simulink model "Tail_sitter_aut1_2016a"  (R2016a)
settings: Solver=ode4  StartTime=0.0  StopTime=13  FixedStep=0.02  RelTol=1e-3
settings Model: Creator=EA-IS  LastModifiedBy=EAIN
settings DebuggingCC: SFUnexpectedBacktrackingDiag=error  SFNoUnconditionalDefaultTransitionDiag=error
settings GRTTargetCC: TargetLangStandard=C99 (ISO)  GeneratePreprocessorConditionals=Use local settings
settings ConfigComp: CovMetricSettings=dwe  CovHtmlReporting=off  CovSaveCumulativeToWorkspaceVar=off  CovSaveSingleToWorkspaceVar=off  CovExternalEMLEnable=on

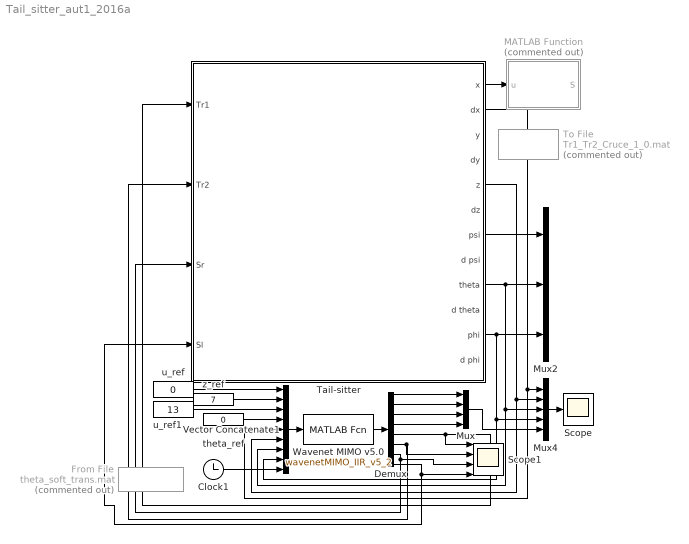
== system Tail_sitter_aut1_2016a ==
  Clock1 : Clock
  Demux : Demux  Outputs=8
  From File : FromFile  Commented=on  FileName=theta_soft_trans.mat  SampleTime=0
  MATLAB Function : MATLAB Function  Commented=on  TreatAsAtomicUnit=on
  Mux : Mux
  Mux2 : Mux  Inputs=3
  Mux4 : Mux  Inputs=5
  Scope : Scope
  Scope1 : Scope  NumInputPorts=4
  "Tail-sitter " : Subsystem
  To File : ToFile  Commented=on  Filename=Tr1_Tr2_Cruce_1_0.mat  SaveFormat=Timeseries
  Vector Concatenate1 : Concatenate  NumInputs=9
  "Wavenet MIMO v5.0 " : MATLABFcn  MATLABFcn=wavenetMIMO_IIR_v5_2  OutputDimensions=8
  theta_ref : Constant  Value=0
  u_ref : Constant  Value=0
  u_ref1 : Constant  Value=13
  z_ref : Constant  Value=7
  wires:
  "Tail-sitter "/7(psi) -> Mux2/1
  Clock1/1 -> Vector Concatenate1/9
  "Tail-sitter "/2(dx) -> Mux4/1, Vector Concatenate1/5
  "Wavenet MIMO v5.0 "/1 -> Demux/1
  "Tail-sitter "/9(theta) -> Mux2/2, Mux4/3, Vector Concatenate1/7
  "Tail-sitter "/11(phi) -> Mux2/3, Mux4/4, Vector Concatenate1/8
  Demux/4 -> Mux/4
  Demux/3 -> Mux/3
  Demux/2 -> Mux/2
  Demux/1 -> Mux/1
  theta_ref/1 -> Vector Concatenate1/4
  "Tail-sitter "/5(z) -> Mux4/2, Vector Concatenate1/6
  z_ref/1 -> Vector Concatenate1/2
  u_ref/1 -> Vector Concatenate1/1
  Mux/1 -> Mux4/5
  Demux/5 -> Scope1/1, "Tail-sitter "/1(Tr1)
  Demux/6 -> Scope1/2, "Tail-sitter "/2("Tr2 ")
  Demux/7 -> Scope1/3, "Tail-sitter "/3(Sr)
  Demux/8 -> Scope1/4, "Tail-sitter "/4("Sl ")
  Vector Concatenate1/1 -> "Wavenet MIMO v5.0 "/1
  u_ref1/1 -> Vector Concatenate1/3
  Mux4/1 -> Scope/1
  "Tail-sitter "/1(x) -> MATLAB Function/1(u)

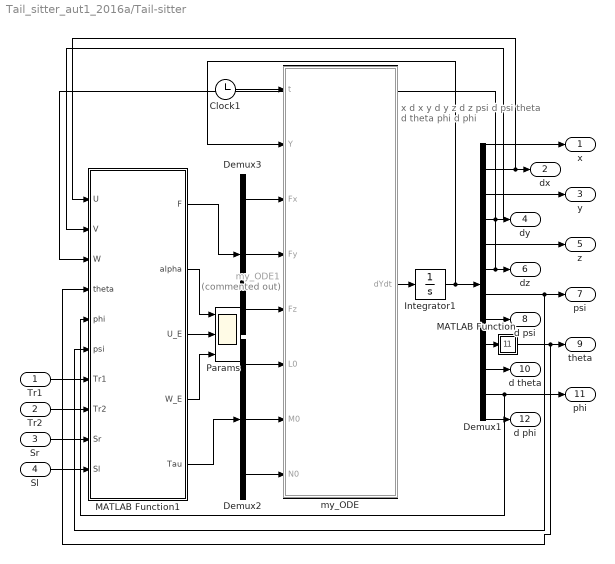
== system Tail_sitter_aut1_2016a/Tail-sitter  ==
  note: x
      |   d x
      |    y
      |   d y
      |    z
      |   d z
      |   psi
      |  d psi
      |  theta
      | d theta
      |   phi
      |  d phi
  Tr1 : Inport
  "Tr2 " : Inport  Port=2
  Sr : Inport  Port=3
  "Sl " : Inport  Port=4
  Clock1 : Clock
  Demux1 : Demux  Outputs=12
  Demux2 : Demux  Outputs=3
  Demux3 : Demux  Outputs=3
  Integrator1 : Integrator  InitialCondition=[0,8.0,0,0,18.0,0,0,0,-pi()/1.97,0,0,0]  UpperSaturationLimit=55  LowerSaturationLimit=-55
  MATLAB Function : MATLAB Function  TreatAsAtomicUnit=on
  MATLAB Function1 : MATLAB Function  TreatAsAtomicUnit=on
  Params : Scope  NumInputPorts=3
  my_ODE : MATLAB Function  TreatAsAtomicUnit=on
  my_ODE1 : MATLAB Function  Commented=on  TreatAsAtomicUnit=on
  x : Outport
  dx : Outport  Port=2
  y : Outport  Port=3
  dy : Outport  Port=4
  z : Outport  Port=5
  dz : Outport  Port=6
  psi : Outport  Port=7
  d psi : Outport  Port=8
  theta : Outport  Port=9
  d theta : Outport  Port=10
  phi : Outport  Port=11
  "d phi " : Outport  Port=12
  wires:
  Demux1/7 -> psi/1, MATLAB Function1/6(psi)
  Demux1/11 -> phi/1, MATLAB Function1/5(phi)
  "Sl "/1 -> MATLAB Function1/10(Sl)
  Demux1/9 -> MATLAB Function/1(theta_rad)
  Demux1/10 -> d theta/1
  Demux1/2 -> MATLAB Function1/1(U), dx/1
  Demux1/8 -> d psi/1
  Demux1/4 -> MATLAB Function1/2(V), dy/1
  Demux1/6 -> MATLAB Function1/3(W), dz/1
  Demux1/3 -> y/1
  Demux1/12 -> "d phi "/1
  Demux1/1 -> x/1
  "Tr2 "/1 -> MATLAB Function1/8(Tr2)
  Sr/1 -> MATLAB Function1/9(Sr)
  Tr1/1 -> MATLAB Function1/7(Tr1)
  Demux1/5 -> z/1
  Demux2/3 -> my_ODE/8(N0)
  Demux2/2 -> my_ODE/7(M0)
  Demux2/1 -> my_ODE/6(L0)
  Demux3/2 -> my_ODE/4(Fy)
  Demux3/1 -> my_ODE/3(Fx)
  Clock1/1 -> my_ODE/1(t)
  my_ODE/1(dYdt) -> Integrator1/1
  Integrator1/1 -> Demux1/1, my_ODE/2(Y)
  Demux3/3 -> my_ODE/5(Fz)
  MATLAB Function1/1(F) -> Demux3/1
  MATLAB Function1/2(alpha) -> Params/1
  MATLAB Function1/3(U_E) -> Params/2
  MATLAB Function1/4(W_E) -> Params/3
  MATLAB Function1/5(Tau) -> Demux2/1
  MATLAB Function/1(theta) -> MATLAB Function1/4(theta), theta/1

== matlab function Tail_sitter_aut1_2016a/MATLAB Function ==
  data: u input; S output
function S = fcn(u)
%S=-40.735;
S=0.4*sin(u)+4;

== matlab function Tail_sitter_aut1_2016a/Tail-sitter /my_ODE ==
  data: t input; dYdt output; Y input; Fx input; Fy input; Fz input; L0 input; M0 input; N0 input
function dYdt = my_ODE(t,Y,Fx,Fy,Fz,L0,M0,N0)
%#codegen

%    This function was generated by the Symbolic Math Toolbox version 8.1.
%    02-Oct-2021 14:11:46

t4 = Y(9);
t2 = cos(t4);
t6 = Y(11);
t3 = cos(t6);
t5 = t2.^2;
t7 = t3.^2;
t8 = sin(t6);
t9 = sin(t4);
t10 = t9.^2;
t11 = t8.^2;
t12 = Y(10);
t13 = Y(12);
t14 = t12.^2;
t15 = Y(8);
t16 = t13.^2;
t17 = t6.*2.0;
t18 = sin(t17);
t19 = t15.^2;
t20 = t7.^2;
t21 = t4.*2.0;
t22 = sin(t21);
t23 = t5.*t20.*4.595542888221475e54;
t24 = t5.*4.407732460960101e54;
t25 = t7.*4.657144927034328e54;
t26 = t10.*5.77375154539186e54;
t27 = t11.*1.244230110983038e49;
t28 = t5.*t7.*t11.*4.595542888221475e54;
t32 = t5.*t7.*9.252684871516254e54;
t33 = t5.*t11.*9.498561560829538e48;
t34 = t7.*t10.*4.657144927034328e54;
t35 = t10.*t11.*1.244230110983038e49;
t29 = t23+t24+t25+t26+t27+t28-t32-t33-t34-t35-5.77375154539186e54;
t30 = 1.0./t29;
t31 = t5.^2;
dYdt = [Y(2);Fx.*(5.0e1./4.9e1);Y(4);Fy.*(5.0e1./4.9e1);Y(6);Fz.*(5.0e1./4.9e1)-9.81e2./1.0e2;t15;t30.*(L0.*3.276779764924493e59-L0.*t7.*2.643071517583136e59-L0.*t11.*7.06138464484666e53+N0.*t9.*3.276779764924493e59-N0.*t2.*t3.*5.32043137111061e56-N0.*t7.*t9.*2.643071517583136e59-N0.*t9.*t11.*7.06138464484666e53-t2.*t8.*t14.*1.919939909312306e55+t2.*t8.*t16.*1.919939909312306e55+t2.*t12.*t13.*1.563784160774438e56-t3.*t12.*t15.*3.839879818624611e55+t9.*t14.*t18.*5.834132374442543e57-t12.*t15.*t22.*9.027036080046288e57+M0.*t2.*t3.*t8.*2.643064456198491e59+N0.*t2.*t3.*t7.*4.291493974897115e56+N0.*t2.*t3.*t11.*4.291493974897115e56+t2.*t7.*t8.*t14.*1.54863581132113e55-t2.*t7.*t8.*t16.*4.137426121757868e49+t2.*t7.*t12.*t13.*2.321039366712225e58-t3.*t8.*t9.*t14.*1.166826474888509e58+t2.*t8.*t11.*t14.*4.137426121757868e49+t3.*t5.*t12.*t15.*3.86527061966559e55+t2.*t7.*t8.*t19.*1.548631673895008e55-t2.*t3.*t14.*t18.*9.472745541356636e54-t2.*t8.*t11.*t16.*4.137426121757868e49+t3.*t7.*t12.*t15.*3.09727162264226e55+t2.*t9.*t12.*t15.*2.349290791384762e58-t2.*t11.*t12.*t13.*3.369918716829444e50+t2.*t8.*t10.*t19.*1.919939909312306e55+t3.*t10.*t12.*t15.*3.839879818624611e55+t3.*t11.*t12.*t15.*8.274852243515736e49-t2.*t12.*t13.*t20.*1.882339395983676e58-t7.*t9.*t14.*t18.*4.705848489959191e57-t9.*t11.*t14.*t18.*1.257242040062484e52+t7.*t12.*t15.*t22.*7.2812650415996e57+t11.*t12.*t15.*t22.*1.945305407657889e52-t2.*t5.*t7.*t8.*t19.*1.20271423951869e55+t3.*t7.*t8.*t9.*t14.*9.411696979918382e57+t3.*t5.*t7.*t12.*t15.*6.713462113741132e54+t2.*t3.*t7.*t14.*t18.*7.640777143974246e54-t3.*t5.*t8.*t9.*t19.*1.166829592250448e58+t3.*t5.*t8.*t13.*t15.*4.387050333958961e57-t2.*t7.*t9.*t12.*t15.*1.894959213772348e58-t2.*t7.*t11.*t12.*t13.*5.028968160249935e52+t3.*t8.*t9.*t11.*t14.*2.514484080124968e52-t2.*t7.*t8.*t10.*t19.*1.54863581132113e55+t3.*t5.*t11.*t12.*t15.*3.076774690411492e55-t2.*t8.*t9.*t13.*t15.*3.839879818624611e55-t3.*t7.*t10.*t12.*t15.*3.09727162264226e55+t2.*t3.*t11.*t14.*t18.*7.640777143974246e54-t2.*t9.*t11.*t12.*t15.*5.06266734741823e52-t2.*t8.*t10.*t11.*t19.*4.137426121757868e49-t3.*t10.*t11.*t12.*t15.*8.274852243515736e49+t2.*t3.*t8.*t19.*t22.*3.640622794272761e57-t2.*t5.*t8.*t19.*t20.*1.528155428794849e55-t3.*t5.*t12.*t15.*t20.*3.056310857589698e55+t2.*t9.*t12.*t15.*t20.*5.028968160249935e52+t3.*t5.*t7.*t8.*t9.*t19.*5.028968160249935e52-t3.*t5.*t7.*t8.*t13.*t15.*5.028968160249935e52-t2.*t5.*t7.*t8.*t11.*t19.*1.528155428794849e55-t3.*t5.*t7.*t11.*t12.*t15.*3.056310857589698e55+t2.*t7.*t8.*t9.*t13.*t15.*8.274852243515736e49+t3.*t5.*t8.*t9.*t11.*t19.*5.028968160249935e52-t3.*t5.*t8.*t11.*t13.*t15.*5.028968160249935e52-t2.*t3.*t8.*t12.*t13.*t18.*9.41167183507758e57+t2.*t7.*t9.*t11.*t12.*t15.*5.028968160249935e52+t2.*t8.*t9.*t11.*t13.*t15.*8.274852243515736e49).*(-4.8828125e-4);t12;t30.*(M0.*2.678494037246015e59-M0.*t5.*2.044785789904658e59-M0.*t10.*2.678494037246015e59+N0.*t8.*4.349008699223577e56+t3.*t16.*1.569390672516609e55+t3.*t19.*1.569390672516609e55+t19.*t22.*3.689424381404189e57+M0.*t5.*t7.*2.643064456198491e59-N0.*t5.*t8.*3.320071303010081e56-N0.*t8.*t10.*4.349008699223577e56-t3.*t5.*t16.*1.198086574525433e55-t3.*t5.*t19.*4.336867919558651e55-t3.*t10.*t16.*1.569390672516609e55-t2.*t13.*t15.*1.920349192777091e58-t3.*t10.*t19.*1.569390672516609e55+t8.*t14.*t18.*7.743179056605651e54-t12.*t13.*t18.*9.537832810566304e57-t5.*t19.*t22.*2.816538862180845e57-t10.*t19.*t22.*3.689424381404189e57+t3.*t19.*t31.*2.396173149050866e55+L0.*t2.*t3.*t8.*2.643064456198491e59+t3.*t5.*t7.*t16.*1.548631673895008e55-t3.*t5.*t11.*t14.*1.548631673895008e55+t3.*t5.*t7.*t19.*1.548631673895008e55+t2.*t5.*t13.*t15.*1.466011380440798e58+t3.*t5.*t11.*t16.*1.548631673895008e55-t2.*t7.*t9.*t19.*9.537832810566304e57+t2.*t7.*t13.*t15.*1.907566562113261e58+t2.*t8.*t12.*t15.*3.118026483837739e55+t3.*t5.*t10.*t19.*3.138781345033217e55-t3.*t5.*t11.*t19.*1.54863581132113e55+t2.*t10.*t13.*t15.*1.920349192777091e58-t3.*t9.*t13.*t15.*3.138781345033217e55+t2.*t9.*t11.*t19.*2.548183267293262e52-t5.*t8.*t14.*t18.*5.911210659223261e54+t5.*t12.*t13.*t18.*7.2812650415996e57-t8.*t10.*t14.*t18.*7.743179056605651e54+t5.*t7.*t19.*t22.*3.640622794272761e57+t10.*t12.*t13.*t18.*9.537832810566304e57-t3.*t7.*t19.*t31.*3.097263347790017e55+t3.*t11.*t19.*t31.*1.182242131844652e55+N0.*t2.*t3.*t8.*t9.*2.643064456198491e59+t3.*t5.*t8.*t12.*t13.*1.261354936560512e56+t2.*t5.*t7.*t9.*t19.*7.2812650415996e57-t2.*t5.*t7.*t13.*t15.*3.351200924701041e58-t2.*t5.*t8.*t12.*t15.*2.380328706370085e55-t2.*t7.*t9.*t11.*t14.*9.41167183507758e57-t2.*t7.*t8.*t12.*t15.*6.194534970432277e55+t3.*t5.*t9.*t13.*t15.*2.396173149050866e55-t2.*t5.*t9.*t11.*t19.*1.945305407657889e52+t2.*t7.*t9.*t10.*t19.*9.537832810566304e57-t2.*t7.*t10.*t13.*t15.*1.907566562113261e58-t2.*t8.*t10.*t12.*t15.*3.118026483837739e55+t3.*t8.*t9.*t12.*t15.*5.096366534586524e52+t3.*t5.*t10.*t11.*t19.*3.097267485216138e55+t3.*t9.*t10.*t13.*t15.*3.138781345033217e55-t2.*t9.*t10.*t11.*t19.*2.548183267293262e52-t2.*t5.*t9.*t19.*t20.*9.41167183507758e57+t2.*t5.*t13.*t15.*t20.*1.882334367015516e58-t5.*t7.*t12.*t13.*t18.*9.41167183507758e57+t3.*t5.*t7.*t8.*t12.*t13.*1.882334367015516e58+t2.*t5.*t7.*t8.*t12.*t15.*8.559010959269338e55-t3.*t5.*t7.*t9.*t13.*t15.*3.097263347790017e55+t3.*t5.*t8.*t9.*t12.*t15.*1.894944025770306e58-t2.*t5.*t7.*t9.*t11.*t19.*9.41167183507758e57+t2.*t5.*t7.*t11.*t13.*t15.*1.882334367015516e58+t2.*t3.*t8.*t9.*t14.*t18.*4.70583591753879e57+t2.*t7.*t8.*t10.*t12.*t15.*6.194534970432277e55-t3.*t5.*t9.*t11.*t13.*t15.*3.097263347790017e55-t3.*t8.*t9.*t10.*t12.*t15.*5.096366534586524e52-t2.*t3.*t8.*t12.*t15.*t22.*7.281245588545523e57).*(-4.8828125e-4);t13;t30.*(N0.*-3.276779764924493e59-L0.*t9.*3.276779764924493e59-M0.*t8.*4.349008699223577e56+N0.*t5.*2.501522350542129e59+N0.*t7.*2.643071517583136e59-t14.*t18.*5.834132374442543e57+L0.*t2.*t3.*5.32043137111061e56+L0.*t7.*t9.*2.643071517583136e59+L0.*t9.*t11.*7.06138464484666e53+M0.*t5.*t8.*3.320071303010081e56+M0.*t8.*t10.*4.349008699223577e56-N0.*t5.*t7.*5.251188970867422e59+N0.*t10.*t11.*7.06138464484666e53+N0.*t5.*t20.*2.608117453284286e59-t3.*t8.*t16.*2.548183267293262e52-t2.*t12.*t15.*2.349290791384762e58-t3.*t8.*t19.*2.548183267293262e52+t5.*t14.*t18.*4.453827714303448e57+t7.*t14.*t18.*4.705848489959191e57-t8.*t19.*t22.*5.990432872627166e54-L0.*t2.*t3.*t7.*4.291493974897115e56-L0.*t2.*t3.*t11.*4.291493974897115e56+N0.*t2.*t3.*t9.*1.064086274222122e57+N0.*t5.*t7.*t11.*2.608117453284286e59-t3.*t5.*t8.*t14.*3.11736193976034e52+t3.*t5.*t8.*t16.*5.06266734741823e52+t2.*t8.*t9.*t14.*1.919939909312306e55+t3.*t5.*t12.*t13.*2.539080104097846e53+t2.*t5.*t12.*t15.*1.793469150865318e58-t2.*t8.*t9.*t16.*1.919939909312306e55+t3.*t5.*t8.*t19.*1.166833516560451e58+t3.*t8.*t10.*t14.*1.166826474888509e58+t2.*t7.*t12.*t15.*4.228599694101606e58-t2.*t9.*t12.*t13.*1.563784160774438e56+t3.*t8.*t10.*t16.*2.548183267293262e52-t2.*t8.*t9.*t19.*1.919939909312306e55+t2.*t8.*t13.*t15.*3.118026483837739e55+t3.*t8.*t10.*t19.*2.548183267293262e52-t5.*t7.*t14.*t18.*9.349463124495094e57-t2.*t12.*t15.*t20.*1.882334367015516e58+t8.*t12.*t13.*t18.*1.54863581132113e55+t10.*t11.*t14.*t18.*1.257242040062484e52+t5.*t8.*t19.*t22.*4.573148882541531e54+t5.*t14.*t18.*t20.*4.643614634535903e57+t9.*t12.*t15.*t22.*9.027036080046288e57+t8.*t10.*t19.*t22.*5.990432872627166e54-t3.*t8.*t19.*t31.*8.907694334715049e57-M0.*t2.*t3.*t8.*t9.*2.643064456198491e59-N0.*t2.*t3.*t7.*t9.*8.582987949794229e56-N0.*t2.*t3.*t9.*t11.*8.582987949794229e56+t3.*t5.*t7.*t8.*t14.*2.514484080124968e52-t3.*t5.*t7.*t8.*t16.*2.514484080124968e52-t2.*t7.*t8.*t9.*t14.*3.443184919592457e55+t3.*t5.*t7.*t12.*t13.*3.768617834016373e55-t2.*t5.*t7.*t12.*t15.*5.546364220221107e58+t3.*t5.*t8.*t11.*t14.*2.514484080124968e52+t2.*t7.*t8.*t9.*t16.*4.137426121757868e49-t3.*t5.*t7.*t8.*t19.*9.411696979918382e57-t3.*t7.*t8.*t10.*t14.*9.411696979918382e57+t2.*t5.*t8.*t9.*t19.*1.465698929861779e55-t2.*t5.*t8.*t13.*t15.*2.380328706370085e55-t2.*t7.*t9.*t12.*t13.*2.321039366712225e58-t3.*t5.*t8.*t11.*t16.*2.514484080124968e52-t2.*t8.*t9.*t11.*t14.*4.137426121757868e49+t3.*t5.*t9.*t12.*t15.*2.880616257641601e55-t3.*t5.*t11.*t12.*t13.*2.048038252628089e53+t2.*t7.*t8.*t9.*t19.*1.548639948747252e55-t2.*t7.*t8.*t13.*t15.*3.09727162264226e55+t3.*t5.*t8.*t10.*t19.*1.138357344934157e52+t2.*t3.*t9.*t14.*t18.*1.894549108271327e55-t2.*t7.*t10.*t12.*t15.*2.333640480329258e58+t2.*t8.*t9.*t11.*t16.*4.137426121757868e49-t3.*t8.*t10.*t11.*t14.*2.514484080124968e52+t2.*t7.*t11.*t12.*t15.*5.028968160249935e52+t2.*t9.*t11.*t12.*t13.*3.369918716829444e50+t2.*t8.*t10.*t13.*t15.*7.218533347868725e54+t3.*t8.*t9.*t13.*t15.*5.096366534586524e52+t2.*t10.*t11.*t12.*t15.*5.06266734741823e52-t3.*t9.*t11.*t12.*t15.*8.274852243515736e49+t2.*t8.*t9.*t14.*t20.*1.528155428794849e55-t3.*t5.*t12.*t13.*t20.*3.056310857589698e55-t2.*t3.*t12.*t15.*t22.*1.465698929861779e55+t2.*t5.*t12.*t15.*t20.*5.609667816760736e58+t5.*t7.*t11.*t14.*t18.*4.643614634535903e57+t2.*t9.*t12.*t13.*t20.*1.882339395983676e58-t5.*t8.*t12.*t13.*t18.*1.182242131844652e55+t2.*t10.*t12.*t15.*t20.*1.882329338047356e58-t8.*t10.*t12.*t13.*t18.*1.54863581132113e55-t7.*t9.*t12.*t15.*t22.*7.2812650415996e57+t3.*t7.*t8.*t19.*t31.*1.869892624899019e58-t9.*t11.*t12.*t15.*t22.*1.945305407657889e52-t3.*t8.*t19.*t20.*t31.*9.287229269071805e57-t2.*t5.*t7.*t8.*t9.*t19.*4.950868240713269e55+t2.*t5.*t7.*t8.*t13.*t15.*6.153582480231959e55+t2.*t7.*t8.*t9.*t11.*t14.*1.528155428794849e55-t3.*t5.*t7.*t9.*t12.*t15.*9.901719931722051e55-t3.*t5.*t7.*t11.*t12.*t13.*3.056310857589698e55+t2.*t5.*t7.*t11.*t12.*t15.*1.869882566962698e58+t3.*t5.*t7.*t8.*t10.*t19.*9.411621545395978e57-t2.*t3.*t7.*t9.*t14.*t18.*1.528155428794849e55-t3.*t5.*t8.*t9.*t13.*t15.*4.387151587305909e57+t2.*t7.*t9.*t11.*t12.*t13.*5.028968160249935e52-t2.*t7.*t8.*t9.*t10.*t19.*1.54863581132113e55+t2.*t7.*t8.*t10.*t13.*t15.*3.097263347790017e55-t3.*t5.*t9.*t11.*t12.*t15.*6.153565930527472e55-t3.*t5.*t8.*t10.*t11.*t19.*7.543452240374903e52-t2.*t3.*t9.*t11.*t14.*t18.*1.528155428794849e55-t2.*t7.*t10.*t11.*t12.*t15.*1.005793632049987e53-t3.*t8.*t9.*t10.*t13.*t15.*5.096366534586524e52+t2.*t8.*t9.*t10.*t11.*t19.*4.137426121757868e49-t2.*t8.*t10.*t11.*t13.*t15.*8.274852243515736e49+t3.*t9.*t10.*t11.*t12.*t15.*8.274852243515736e49+t2.*t3.*t7.*t12.*t15.*t22.*1.182242131844652e55-t2.*t5.*t7.*t12.*t15.*t20.*1.857445853814361e58-t2.*t3.*t8.*t9.*t19.*t22.*3.640622794272761e57+t2.*t5.*t8.*t9.*t19.*t20.*4.584466286384548e55-t2.*t5.*t8.*t13.*t15.*t20.*3.056310857589698e55+t3.*t5.*t9.*t12.*t15.*t20.*6.112621715179397e55+t2.*t3.*t11.*t12.*t15.*t22.*1.182242131844652e55-t2.*t5.*t11.*t12.*t15.*t20.*1.857445853814361e58-t3.*t7.*t8.*t11.*t19.*t31.*9.287229269071805e57+t3.*t5.*t7.*t8.*t9.*t13.*t15.*1.005793632049987e53+t2.*t5.*t7.*t8.*t9.*t11.*t19.*4.584466286384548e55-t2.*t5.*t7.*t8.*t11.*t13.*t15.*3.056310857589698e55+t3.*t5.*t7.*t9.*t11.*t12.*t15.*6.112621715179397e55+t3.*t5.*t8.*t9.*t11.*t13.*t15.*1.005793632049987e53+t2.*t3.*t8.*t9.*t12.*t13.*t18.*9.41167183507758e57).*4.8828125e-4];

== matlab function Tail_sitter_aut1_2016a/Tail-sitter /MATLAB Function1 ==
  data: F output; alpha output; U_E output; W_E output; U input; V input; W input; theta input; phi input; psi input; Tr1 input; Tr2 input; Sr input; Sl input; Tau output
function [F, alpha,   U_E, W_E,  Tau]=Forces1_1(U, V, W, theta, phi, psi, Tr1, Tr2, Sr, Sl)
%%%%%%%%%%%%%%%%%ASUMIENDO  HOVER%%%%%%%%%%%%%%%%%
f1=Motor(Tr1); f2=Motor(Tr2); l=0.2;%syms f1 f2 TauMi1 TauMi2 Sr Sl; %Parámetros de motores
u=f1(1)+f2(1);   %Vector de fuerzas de motores
F_barMotors=[0; 0; u];  %Fuerzas que contribuyen a la tracción en el eje z
Tau_Motors=[f1(2)-f2(2);0;(f2(1)-f1(1))*l]; coder.extrinsic('assignin');
 %%%%%%%%%%%%%ASUMIENDO MARCO VUELO CRUCERO%%%%%%%%%%%%%%%%%%%
 R_be=[cos(theta)*cos(psi) cos(theta)*sin(psi) -sin(theta);
     -cos(phi)*sin(psi)+sin(phi)*sin(theta)*cos(psi) cos(phi)*cos(psi)+sin(phi)*sin(theta)*sin(psi) sin(phi)*cos(theta);
     sin(phi)*sin(psi)+cos(phi)*sin(theta)*cos(psi) -sin(phi)*cos(psi)+cos(phi)*sin(theta)*sin(psi) cos(phi)*cos(theta)];
 if W==0
    W=0.01; 
 end
VT= min(19, max(0, norm([U V W])));
if VT<0.1
   aerofact=0;
else
    aerofact=1;
end
Vel_rotated=R_be*[filter((1/1)*ones(1,1),19,U);V;filter((1/1)*ones(1,1),19,W)];
U_E=Vel_rotated(1); W_E=Vel_rotated(3);
alpha=filter((1/1)*ones(1,1),19,rad2deg(atan(Vel_rotated(1)/Vel_rotated(3)))); beta=0;
%assignin('base','alpha',alpha);
%alpha=6; beta=0; %VT=3;
q=1/2*0.9691*(VT^2); S=0.00493782; %Constantes físicas
[CL, CD, CY, Cl, Cm, Cn]=Aero_Coefs1(alpha, beta, Sr, Sl); %Función donde se calculan los coeficientes aerodinámicos
Lift=(CL)*q*S; %Fuerza de levantamiento
Drag=(CD)*q*S; %Fuerza de arrastre
Fay=(CY)*q*S;  %Fuerza lateral
%assignin('base','Drag',Drag);
%assignin('base','Lift',Lift);
%assignin('base','alpha',alpha); assignin('base','Sl',Sl); assignin('base','VT',VT);
%F_barWing=[-1*(Drag*sin(deg2rad(alpha))+Lift*cos(deg2rad(alpha)));Fay;1*(-Drag*cos(deg2rad(alpha))+Lift*sin(deg2rad(alpha)))];
%F_barWing=[-1*(Drag*cos(deg2rad(alpha))+Lift*sin(deg2rad(alpha)));Fay;1*(-Drag*sin(deg2rad(alpha))+Lift*cos(deg2rad(alpha)))];
F_barWing=[-Lift*cos(deg2rad(alpha))+Drag*sin(deg2rad(alpha));Fay;-Lift*sin(deg2rad(alpha))-Drag*cos(deg2rad(alpha))]; 
Lbar=(Cl)*q*S*(1); %(Cl)*q*S*b;
Mbar=(Cm)*q*S*(1); %(Cm)*q*S*MAC;
Nbar=(Cn)*q*S*(1); %(Cn)*q*S*b;
Tau_Wing=[0*Nbar; 1*Mbar; 0*Lbar];  % Inversión de variables en el vector
%%%%%%%%%%%%%%%%%%%%%%%%%%%%%VALORES TOTALES%%%%%%%%%%%%%%%%%%%%%%%%%%%%%%%%
F_tot=aerofact*F_barWing+F_barMotors; Tau=Tau_Motors+aerofact*Tau_Wing; %Tau=filter((1/1)*ones(1,1),16,Tau_Motors+aerofact*Tau_Wing);
 F=R_be*F_tot; %Fueerzas totales rotadas
 %assignin('base','F',F);

== matlab function Tail_sitter_aut1_2016a/Tail-sitter /my_ODE1 ==
  data: t input; dYdt output; Y input; Fx input; Fy input; Fz input; L0 input; M0 input; N0 input
function dYdt = my_ODE(t,Y,Fx,Fy,Fz,L0,M0,N0)
%#codegen

%    This function was generated by the Symbolic Math Toolbox version 8.1.
%    16-Aug-2021 19:45:59

t4 = Y(9);
t2 = cos(t4);
t6 = Y(11);
t3 = cos(t6);
t5 = t2.^2;
t7 = t3.^2;
t8 = sin(t4);
t9 = t8.^2;
t10 = sin(t6);
t11 = Y(8);
t12 = Y(10);
t13 = Y(12);
t14 = t7.^2;
t15 = t4.*2.0;
t16 = sin(t15);
t17 = t10.^2;
t18 = t5.*t14.*1.170455833668586e31;
t19 = t5.*1.1226187013002e31;
t20 = t7.*1.186142316045941e31;
t21 = t9.*1.470534230225482e31;
t22 = t5.*t7.*t17.*1.170455833668586e31;
t26 = t5.*t7.*2.356598149714528e31;
t27 = t7.*t9.*1.186142316045941e31;
t23 = t18+t19+t20+t21+t22-t26-t27-1.470534230225482e31;
t24 = 1.0./t23;
t25 = t11.^2;
t28 = t12.^2;
t29 = t5.^2;
dYdt = [Y(2);Fx;Y(4);Fy;Y(6);Fz-1.5696e1;t11;-t24.*(L0.*2.546914493532914e32-L0.*t7.*2.05435752125735e32+N0.*t8.*2.546914493532914e32-N0.*t7.*t8.*2.05435752125735e32+t2.*t12.*t13.*1.944750556124309e29-t11.*t12.*t16.*1.1226187013002e31+M0.*t2.*t3.*t10.*2.05435752125735e32+t2.*t8.*t11.*t12.*2.921620954889721e31+t2.*t7.*t12.*t13.*2.886486966951123e31-t2.*t12.*t13.*t14.*2.340911667337173e31+t7.*t11.*t12.*t16.*9.055114250502889e30-t2.*t7.*t8.*t11.*t12.*2.356598149714528e31+t3.*t5.*t10.*t11.*t13.*5.4557529961395e30-t2.*t7.*t12.*t13.*t17.*2.340911667337173e31-t3.*t5.*t8.*t10.*t25.*5.4557529961395e30);t12;t24.*(M0.*1.873701071275537e33-M0.*t5.*1.43039979622753e33-M0.*t9.*1.873701071275537e33+M0.*t5.*t7.*1.848921769131615e33-t2.*t11.*t13.*2.149363210637046e32+t2.*t8.*t25.*8.25882403434112e31+L0.*t2.*t3.*t10.*1.848921769131615e33+t2.*t5.*t11.*t13.*1.640842685979372e32+t2.*t7.*t11.*t13.*2.135056168882694e32+t2.*t9.*t11.*t13.*2.149363210637046e32-t3.*t10.*t12.*t13.*2.135056168882694e32-t2.*t5.*t8.*t25.*6.304858548091923e31-t2.*t7.*t8.*t25.*1.067528084441347e32-t2.*t8.*t9.*t25.*8.25882403434112e31+N0.*t2.*t3.*t8.*t10.*1.848921769131615e33-t2.*t5.*t7.*t11.*t13.*3.750858899833595e32-t2.*t7.*t9.*t11.*t13.*2.135056168882694e32+t3.*t5.*t10.*t12.*t13.*1.644038399230139e32+t2.*t5.*t11.*t13.*t14.*2.106820500603456e32+t2.*t5.*t7.*t8.*t25.*1.62992056509052e32+t3.*t9.*t10.*t12.*t13.*2.135056168882694e32+t2.*t7.*t8.*t9.*t25.*1.067528084441347e32-t2.*t5.*t8.*t14.*t25.*1.053410250301728e32+t3.*t5.*t8.*t10.*t11.*t12.*2.120938334743075e32-t2.*t3.*t10.*t11.*t12.*t16.*8.1496028254526e31+t2.*t5.*t7.*t11.*t13.*t17.*2.106820500603456e32-t2.*t5.*t7.*t8.*t17.*t25.*1.053410250301728e32).*(-1.0./9.0);t13;t24.*(N0.*2.649078964511616e48+L0.*t8.*2.649078964511616e48-N0.*t5.*2.022330065941892e48-N0.*t7.*2.136764037021151e48-L0.*t7.*t8.*2.136764037021151e48+N0.*t5.*t7.*4.245269819566539e48-N0.*t5.*t14.*2.108505782545388e48+t2.*t11.*t12.*3.038816039379016e47+t3.*t10.*t28.*1.509294217670373e47-N0.*t5.*t7.*t17.*2.108505782545388e48-t2.*t5.*t11.*t12.*2.319858759829617e47-t2.*t7.*t11.*t12.*5.469716889816706e47+t2.*t8.*t12.*t13.*2.022760403826882e45+t2.*t11.*t12.*t14.*2.434812739677309e47-t3.*t5.*t10.*t25.*1.509294217670373e47-t3.*t5.*t10.*t28.*1.152208414938572e47-t8.*t11.*t12.*t16.*1.167650344891045e47-t3.*t7.*t10.*t28.*1.217406369838654e47-t3.*t9.*t10.*t28.*1.509294217670373e47+t3.*t10.*t25.*t29.*1.152208414938572e47+M0.*t2.*t3.*t8.*t10.*2.136764037021151e48+t2.*t5.*t7.*t11.*t12.*7.174258081124561e47+t2.*t7.*t9.*t11.*t12.*3.018588435340747e47+t2.*t7.*t8.*t12.*t13.*3.002272720542096e47-t2.*t5.*t11.*t12.*t14.*7.256138390314372e47-t2.*t9.*t11.*t12.*t14.*2.434812739677309e47-t2.*t8.*t12.*t13.*t14.*2.434812739677309e47+t3.*t5.*t7.*t10.*t25.*1.217406369838654e47+t3.*t5.*t9.*t10.*t25.*9.418342368055859e46+t3.*t5.*t7.*t10.*t28.*2.418712796771457e47+t7.*t8.*t11.*t12.*t16.*9.418342368055859e46+t3.*t7.*t9.*t10.*t28.*1.217406369838654e47-t3.*t5.*t10.*t14.*t28.*1.201306426932803e47-t3.*t7.*t10.*t25.*t29.*2.418712796771457e47+t3.*t10.*t14.*t25.*t29.*1.201306426932803e47+t3.*t5.*t8.*t10.*t11.*t13.*5.674599808647875e46+t2.*t5.*t7.*t11.*t12.*t14.*2.402612853865606e47-t2.*t5.*t7.*t11.*t12.*t17.*2.418712796771457e47-t2.*t7.*t8.*t12.*t13.*t17.*2.434812739677309e47-t3.*t5.*t7.*t9.*t10.*t25.*1.217406369838654e47+t2.*t5.*t11.*t12.*t14.*t17.*2.402612853865606e47-t3.*t5.*t7.*t10.*t17.*t28.*1.201306426932803e47+t3.*t7.*t10.*t17.*t25.*t29.*1.201306426932803e47).*(-9.61433965409356e-17)];

== matlab function Tail_sitter_aut1_2016a/Tail-sitter /MATLAB Function ==
  data: theta_rad input; theta output
function theta = fcn(theta_rad)
%#codegen
theta_norma = mod(theta_rad, 2*pi);

if theta_norma > pi
    theta_norma = theta_norma - 2*pi;
else
    theta_norma = mod(theta_rad, 2*pi);
end
theta = theta_norma;
